simulink model "simu"  (Simulink 7.5)
settings: Solver=ode4  StartTime=0.0  StopTime=tf  FixedStep=dt  RelTol=1e-3
values from neighbouring files (symbols this model uses):
  a0 = 4    [delta_calc.m]
  s0 = 0    [delta_calc.m]
  v0 = 10    [delta_calc.m]
settings Model: Creator=Administrator  LastModifiedBy=Administrator

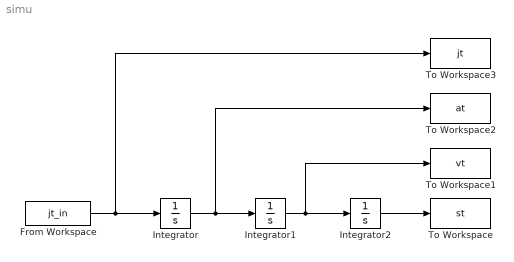
== system simu ==
  From Workspace : FromWorkspace  VariableName=jt_in  SampleTime=0
  Integrator : Integrator  InitialCondition=a0
  Integrator1 : Integrator  InitialCondition=v0
  Integrator2 : Integrator  InitialCondition=s0
  To Workspace : ToWorkspace  VariableName=st  SampleTime=-1  SaveFormat=Array
  To Workspace1 : ToWorkspace  VariableName=vt  SampleTime=-1  SaveFormat=Array
  To Workspace2 : ToWorkspace  VariableName=at  SampleTime=-1  SaveFormat=Array
  To Workspace3 : ToWorkspace  VariableName=jt  SampleTime=-1  SaveFormat=Array
  wires:
  Integrator/1 -> Integrator1/1, To Workspace2/1
  Integrator1/1 -> Integrator2/1, To Workspace1/1
  Integrator2/1 -> To Workspace/1
  From Workspace/1 -> Integrator/1, To Workspace3/1
